simulink model "expiriment_dynamic_target"  (R2024b)
settings: Solver=VariableStepAuto  StartTime=0.0  StopTime=50.0  RelTol=1e-3
settings Model: Creator=Omer Mizrachi  LastModifiedBy=alonorlicky

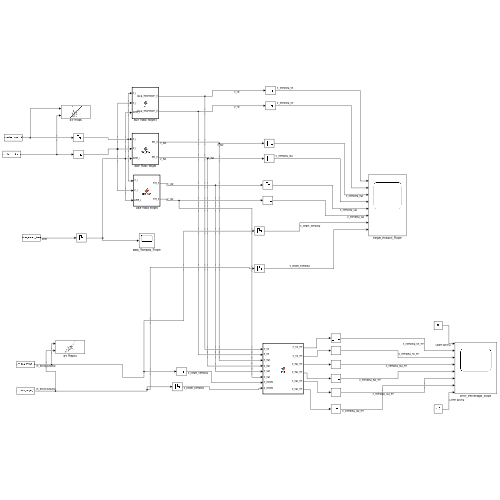
[thumbnail: Simulink's stored preview of the top-level diagram]
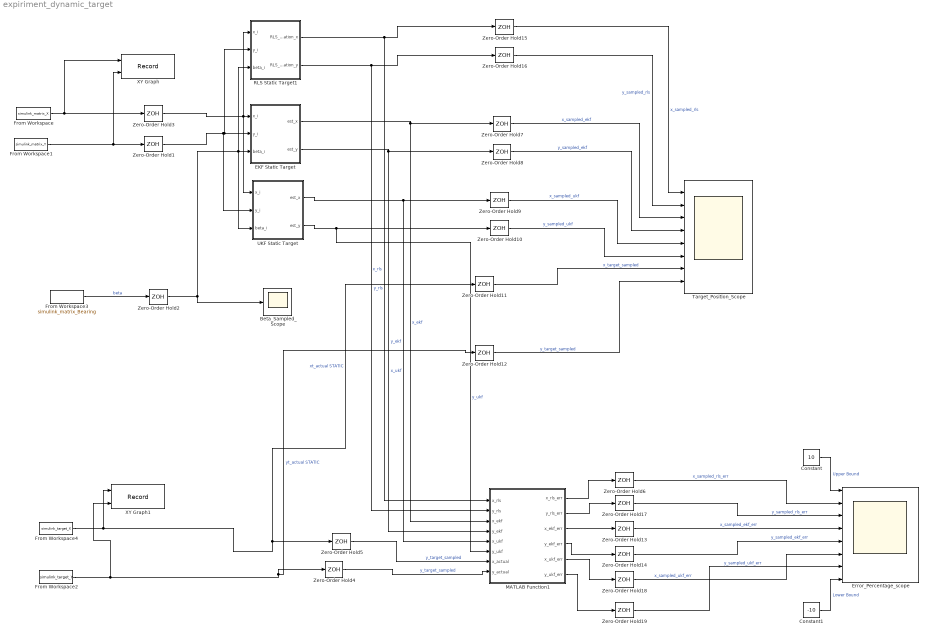
== system expiriment_dynamic_target ==
  Beta_Sampled_Scope : Scope
  Constant : Constant  Value=10
  Constant1 : Constant  Value=-10
  EKF Static Target : MATLAB Function  TreatAsAtomicUnit=on
  Error_Percentage_scope : Scope  NumInputPorts=8
  From Workspace : FromWorkspace  VariableName=simulink_matrix_X
  From Workspace1 : FromWorkspace  VariableName=simulink_matrix_Y
  From Workspace2 : FromWorkspace  VariableName=simulink_target_Y
  From Workspace3 : FromWorkspace  VariableName=simulink_matrix_Bearing
  From Workspace4 : FromWorkspace  VariableName=simulink_target_X
  MATLAB Function1 : MATLAB Function  TreatAsAtomicUnit=on
  RLS Static Target1 : MATLAB Function  TreatAsAtomicUnit=on
  Target_Position_Scope : Scope  NumInputPorts=8
  UKF Static Target : MATLAB Function  TreatAsAtomicUnit=on
  XY Graph : Record  FileSettingsInternal="{\"entries\":[{\"content\":{\"excelSettings\":{\"content\":{},\"type\":\"Streamout.ExcelSettings\"}},\"type\":\"Streamout.FileSettingStorage\",\"uuid\":\"\"}],\"packageUris\":[\"http:\\/\\/schema.mathworks.com\\/mf0\\/streamout_blocks\\/R2020a\"],\"version\":\"1.0\"}"  Layout=[1 1]  SignalsInternal="{\"entries\":[{\"content\":{\"signals\":[{\"content\":{\"blockPath\":[],\"dimensions\":[1],\"domain\":\"\",\"lineColor\":\"#0072bd\",\"lineWidth\":2,\"plots\":[ 1 ],\"port\":1,\"sid\":[\"\"],\"signalID\":1,\"signalName\":\"From\\nWorkspace\"},\"type\":\"RecordBlkView.Signal\",\"uuid\":\"\"},{\"content\":{\"blockPath\":[],\"dimensions\":[1],\"domain\":\"\",\"lineColor\":\"#d95319\",\"lineWidth\":2,\"plots\":[ 1 ],\"port\":2,\"sid\":[\"\"],\"signalID\":2,\"signalName\":\"From\\nWorkspace1\"},\"type\":\"RecordBlkView.Signal\",\"uuid\":\"\"}]},\"type\":\"RecordBlkView.InputSignals\",\"uuid\":\"\"}],\"packageUris\":[\"http:\\/\\/schema.mathworks.com\\/mf0\\/streamout_blocks\\/R2020a\"],\"version\":\"1.0\"}"  VisualizationBindings="{\"xyplotplugin\":{\"info\":[{\"series\":[{\"bindingParametersList\":[{\"parameter\":\"X-Axis\",\"signalID\":1,\"signalName\":\"From\\nWorkspace\"},{\"parameter\":\"Y-Axis\",\"signalID\":2,\"signalName\":\"From\\nWorkspace1\"}],\"seriesID\":0}],\"subplotID\":1}]}}"  CompatibilityTag=XY
  XY Graph1 : Record  FileSettingsInternal="{\"entries\":[{\"content\":{\"excelSettings\":{\"content\":{},\"type\":\"Streamout.ExcelSettings\"}},\"type\":\"Streamout.FileSettingStorage\",\"uuid\":\"\"}],\"packageUris\":[\"http:\\/\\/schema.mathworks.com\\/mf0\\/streamout_blocks\\/R2020a\"],\"version\":\"1.0\"}"  Layout=[1 1]  SignalsInternal="{\"entries\":[{\"content\":{\"signals\":[{\"content\":{\"blockPath\":[],\"dimensions\":[1],\"domain\":\"\",\"lineColor\":\"#0072bd\",\"lineWidth\":2,\"plots\":[ 1 ],\"port\":1,\"sid\":[\"\"],\"signalID\":1,\"signalName\":\"xt_actual STATIC\"},\"type\":\"RecordBlkView.Signal\",\"uuid\":\"\"},{\"content\":{\"blockPath\":[],\"dimensions\":[1],\"domain\":\"\",\"lineColor\":\"#d95319\",\"lineWidth\":2,\"plots\":[ 1 ],\"port\":2,\"sid\":[\"\"],\"signalID\":2,\"signalName\":\"yt_actual STATIC\"},\"type\":\"RecordBlkView.Signal\",\"uuid\":\"\"}]},\"type\":\"RecordBlkView.InputSignals\",\"uuid\":\"\"}],\"packageUris\":[\"http:\\/\\/schema.mathworks.com\\/mf0\\/streamout_blocks\\/R2020a\"],\"version\":\"1.0\"}"  VisualizationBindings="{\"xyplotplugin\":{\"info\":[{\"series\":[{\"bindingParametersList\":[{\"parameter\":\"X-Axis\",\"signalID\":1,\"signalName\":\"xt_actual STATIC\"},{\"parameter\":\"Y-Axis\",\"signalID\":2,\"signalName\":\"yt_actual STATIC\"}],\"seriesID\":0}],\"subplotID\":1}]}}"  CompatibilityTag=XY
  Zero-Order Hold{1..19} (19 alike) : ZeroOrderHold  SampleTime=0.01
  wires:
  From Workspace1/1 -> XY Graph/2, Zero-Order Hold1/1
  From Workspace/1 -> XY Graph/1, Zero-Order Hold3/1
  Zero-Order Hold2/1 -> Beta_Sampled_Scope/1, UKF Static Target/3(beta_i), RLS Static Target1/3(beta_i), EKF Static Target/3(beta_i)
  From Workspace3/1 -> Zero-Order Hold2/1  "beta"
  Zero-Order Hold3/1 -> UKF Static Target/1(x_i), RLS Static Target1/1(x_i), EKF Static Target/1(x_i)
  Zero-Order Hold1/1 -> UKF Static Target/2(y_i), RLS Static Target1/2(y_i), EKF Static Target/2(y_i)
  From Workspace2/1 -> XY Graph1/2, Zero-Order Hold12/1, Zero-Order Hold4/1  "yt_actual STATIC"
  From Workspace4/1 -> XY Graph1/1, Zero-Order Hold11/1, Zero-Order Hold5/1  "xt_actual STATIC"
  Zero-Order Hold4/1 -> MATLAB Function1/8(y_actual)  "y_target_sampled"
  Zero-Order Hold5/1 -> MATLAB Function1/7(x_actual)  "y_target_sampled"
  RLS Static Target1/1(RLS_estimation_x) -> MATLAB Function1/1(x_rls), Zero-Order Hold15/1  "x_rls"
  Zero-Order Hold8/1 -> Target_Position_Scope/4  "y_sampled_ekf"
  RLS Static Target1/2(RLS_estimation_y) -> MATLAB Function1/2(y_rls), Zero-Order Hold16/1  "y_rls"
  Zero-Order Hold10/1 -> Target_Position_Scope/6  "y_sampled_ukf"
  Zero-Order Hold11/1 -> Target_Position_Scope/7  "x_target_sampled"
  EKF Static Target/1(est_x) -> MATLAB Function1/3(x_ekf), Zero-Order Hold7/1  "x_ekf"
  UKF Static Target/1(est_x) -> MATLAB Function1/5(x_ukf), Zero-Order Hold9/1  "x_ukf"
  Zero-Order Hold12/1 -> Target_Position_Scope/8  "y_target_sampled"
  Zero-Order Hold9/1 -> Target_Position_Scope/5  "x_sampled_ukf"
  Zero-Order Hold7/1 -> Target_Position_Scope/3  "x_sampled_ekf"
  EKF Static Target/2(est_y) -> MATLAB Function1/4(y_ekf), Zero-Order Hold8/1  "y_ekf"
  Zero-Order Hold16/1 -> Target_Position_Scope/2  "y_sampled_rls"
  Zero-Order Hold15/1 -> Target_Position_Scope/1  "x_sampled_rls"
  UKF Static Target/2(est_y) -> MATLAB Function1/6(y_ukf), Zero-Order Hold10/1  "y_ukf"
  Zero-Order Hold14/1 -> Error_Percentage_scope/5  "y_sampled_ekf_err"
  MATLAB Function1/6(y_ukf_err) -> Zero-Order Hold19/1
  Zero-Order Hold13/1 -> Error_Percentage_scope/4  "x_sampled_ekf_err"
  Zero-Order Hold19/1 -> Error_Percentage_scope/7  "y_sampled_ukf_err"
  Zero-Order Hold18/1 -> Error_Percentage_scope/6  "x_sampled_ukf_err"
  MATLAB Function1/5(x_ukf_err) -> Zero-Order Hold18/1
  Constant/1 -> Error_Percentage_scope/1  "Upper Bound"
  Zero-Order Hold6/1 -> Error_Percentage_scope/2  "x_sampled_rls_err"
  MATLAB Function1/2(y_rls_err) -> Zero-Order Hold17/1
  Constant1/1 -> Error_Percentage_scope/8  "Lower Bound"
  MATLAB Function1/4(y_ekf_err) -> Zero-Order Hold14/1
  Zero-Order Hold17/1 -> Error_Percentage_scope/3  "y_sampled_rls_err"
  MATLAB Function1/1(x_rls_err) -> Zero-Order Hold6/1
  MATLAB Function1/3(x_ekf_err) -> Zero-Order Hold13/1

== matlab function expiriment_dynamic_target/RLS Static Target1 ==
  data: x_i input; RLS_estimation_x output; y_i input; beta_i input; RLS_estimation_y output
function [RLS_estimation_x, RLS_estimation_y] = fcn(x_i, y_i, beta_i)
% fcn - Recursive Least Squares estimator for 2D static target

    % Persistent variables
    persistent covarience_matrix state_estimate

    % RLS parameter
    lambda = 1;

    % Initialization 
    if isempty(covarience_matrix)
        covarience_matrix = eye(2);  % Initial covariance matrix
    end

    if isempty(state_estimate)
        state_estimate = zeros(2, 1);  % Initial position estimate [0; 0]
    end

    % Compute direction vector (orthogonal to bearing)
    direction_vector = [-sin(beta_i); cos(beta_i)];

    % Project measurement to direction vector
    z_i = y_i * cos(beta_i) - x_i * sin(beta_i);

    % Compute innovation (measurement residual)
    innovation = z_i - direction_vector' * state_estimate;

    % Update state estimate
    gain_denominator = lambda + direction_vector' * covarience_matrix * direction_vector;
    gain_numerator   = covarience_matrix * direction_vector;
    state_estimate   = state_estimate + (gain_numerator / gain_denominator) * innovation;

    % Update covariance matrix
    gain_vector        = covarience_matrix * direction_vector / (1 + direction_vector' * covarience_matrix * direction_vector);
    covarience_matrix  = covarience_matrix - gain_vector * direction_vector' * covarience_matrix;

    % Output estimated position
    RLS_estimation_x = state_estimate(1);
    RLS_estimation_y = state_estimate(2);
end

== matlab function expiriment_dynamic_target/MATLAB Function1 ==
  data: x_rls input; y_rls input; x_rls_err output; y_rls_err output; x_ekf input; x_ekf_err output; y_ekf input; x_ukf input; y_ukf input; x_actual input; y_actual input; y_ekf_err output; x_ukf_err output; y_ukf_err output
function [x_rls_err,y_rls_err,x_ekf_err,y_ekf_err,x_ukf_err,y_ukf_err]= fcn(x_rls,y_rls,x_ekf,y_ekf,x_ukf,y_ukf,x_actual,y_actual)

x_rls_err = ((x_rls - x_actual)/x_actual)*100;
y_rls_err = ((y_rls - y_actual)/y_actual)*100;

x_ekf_err = ((x_ekf - x_actual)/x_actual)*100;
y_ekf_err = ((y_ekf - y_actual)/y_actual)*100;

x_ukf_err = ((x_ukf - x_actual)/x_actual)*100;
y_ukf_err = ((y_ukf - y_actual)/y_actual)*100;

== matlab function expiriment_dynamic_target/UKF Static Target ==
  data: x_i input; est_x output; y_i input; beta_i input; est_y output
function [est_x, est_y] = ukf_fcn(x_i, y_i, beta_i)

persistent X_i P Q R lambda alpha beta nx


if isempty(P)
    nx = 6;
    P = 1000* eye(nx);
    Q = 0.001 * diag([0.01, 0.01, 1, 0.01, 1, 0.01]);
    R = diag([1, 1, 100]);
    
    alpha = 1e-3;
    beta = 2;
    lambda = alpha^2 * (nx + 1) - nx;
end

if isempty(X_i)
    X_i = zeros(nx, 1);
end

dt = 0.01;

Wm = [lambda / (nx + lambda); repmat(1 / (2 * (nx + lambda)), 2 * nx, 1)];
Wc = Wm;
Wc(1) = Wc(1) + (1 - alpha^2 + beta);

sigma_points = generate_sigma_points(X_i, P, lambda);

predicted_sigma_points = process_model(sigma_points, dt);
[X_pred, P_pred] = compute_mean_and_covariance(predicted_sigma_points, Wm, Wc, Q);

measured_sigma_points = measurement_model(predicted_sigma_points, beta_i);
[y_pred, Pyy] = compute_mean_and_covariance(measured_sigma_points, Wm, Wc, R);

Pxy = compute_cross_covariance(predicted_sigma_points, measured_sigma_points, X_pred, y_pred, Wc);

K = Pxy / Pyy;

meas = [x_i; y_i; 0];
resid = meas - y_pred;
X_i = X_pred + K * resid;
P = P_pred - K * Pyy * K';

est_x = X_i(1);
est_y = X_i(2);

end

%% Helper Functions

function sigma_points = generate_sigma_points(mean, covariance, lambda)
    nx = length(mean);
    S = chol((nx + lambda) * covariance, 'lower');
    sigma_points = [mean, bsxfun(@plus, mean, S), bsxfun(@minus, mean, S)];
end

function predicted_sigma_points = process_model(sigma_points, dt)
    F = [1 0 0 0 0 0;
         0 1 0 0 0 0;
         0 0 1 dt 0 0;
         0 0 0 1 0 0;
         0 0 0 0 1 dt;
         0 0 0 0 0 1];
    predicted_sigma_points = F * sigma_points;
end

function measured_sigma_points = measurement_model(sigma_points, beta_i)
    H = [0 0 1 0 0 0;
         0 0 0 0 1 0;
         sin(beta_i) -cos(beta_i) -sin(beta_i) 0 cos(beta_i) 0];
    measured_sigma_points = H * sigma_points;
end

function [mean_out, covariance] = compute_mean_and_covariance(sigma_points, Wm, Wc, noise_cov)
    mean_out = sigma_points * Wm;
    diff = bsxfun(@minus, sigma_points, mean_out);
    covariance = diff * diag(Wc) * diff' + noise_cov;
end

function Pxy = compute_cross_covariance(predicted_sigma_points, measured_sigma_points, X_pred, y_pred, Wc)
    diff_x = bsxfun(@minus, predicted_sigma_points, X_pred);
    diff_y = bsxfun(@minus, measured_sigma_points, y_pred);
    Pxy = diff_x * diag(Wc) * diff_y';
end

== matlab function expiriment_dynamic_target/EKF Static Target ==
  data: x_i input; est_x output; y_i input; beta_i input; est_y output
function [est_x, est_y] = ekf_fcn(x_i, y_i, beta_i)

persistent X_i P Q R

if isempty(P)
    P = 1000*eye(6);
    Q = 0.01*diag([0.001, 0.001, 0.1, 0.001, 0.1, 0.001]);
    R = diag([1, 1, 200]);
end

if isempty(X_i)
    X_i = zeros(6, 1);
end

dt = 0.01;

F = [1 0 0 0 0 0 ;
     0 1 0 0 0 0 ; 
     0 0 1 dt 0 0; 
     0 0 0 1 0 0 ; 
     0 0 0 0 1 dt; 
     0 0 0 0 0 1];

H = [0 0 1 0 0 0 ; 
     0 0 0 0 1 0 ; 
    sin(beta_i) -cos(beta_i) -sin(beta_i) 0 cos(beta_i) 0];

X_i = F*X_i;
measurement = [x_i ; y_i ; 0];
predicted_measurement = H*X_i;
P = F*P*F' + Q;
innovation = measurement - predicted_measurement;
K = P*H'/(H*P*H' + R);
X_i = X_i + K*innovation;
P = (eye(6) - K*H)*P;
est_x = X_i(1);
est_y = X_i(2);

end
